simulink model "affine_single_integrator_ex"  (R2020b)
settings: Solver=ode4  StartTime=0.0  StopTime=50  FixedStep=0.01  RelTol=1e-3
InitFcn:
  | Initial_Parameters;
values from neighbouring files (symbols this model uses):
  cmd_sample = 0.1    [run_by_script.m]
  delay = 0.01    [Initial_Parameters.m]    (also in run_by_script.m)
  kalpha = 0.5    [Initial_Parameters.m]    (also in run_by_script.m)
  kbeta = 1.5    [Initial_Parameters.m]    (also in run_by_script.m = 0.5)
  kptheta = 100    [run_by_script.m]
  Kv = 0.987 / Tv    (= 6.16875)    [run_by_script.m]
  L = 10.5e-3    (= 0.0105)    [run_by_script.m]
  noise_p = normrnd(0.001, 0.03,[1 6])    [run_by_script.m]
  noise_pT = 3    [run_by_script.m]
  noise_v = normrnd(0.001, 0.03,[1 6])    [run_by_script.m]
  noise_vT = 0.1    [run_by_script.m]
  p = p(tout >= start_time, :)    [read_data.m]
  P0 = [2 0 ... (first row only)    [Initial_Parameters.m]    (also in run_by_script.m = [p(1,1:2:end)' p(2,2:2:end)'])
  R = 3.2e-3    (= 0.0032)    [run_by_script.m]
  seed_p = zeros(1,6)    [run_by_script.m]
  seed_v = zeros(1,6)    [run_by_script.m]
  stressMat = -fcn_StressMatrix(2,nodenum,m,P,neighborMat,fig_shape)    [Initial_Parameters.m]    (also in fcn_StressMatrix.m = -stressMat)
  tout = tout(tout >= start_time) - start_time    [read_data.m]    (also in run_by_script.m = out.tout)
  Tv = 0.16    [run_by_script.m]
  vl = 1    [run_by_script.m]
libraries: simulink x24
settings Model: Creator=Fitz  LastModifiedBy=xpp
settings OptimizationCC: BlockReduction=off  DefaultParameterBehavior=Inlined  BufferReuse=off
settings DebuggingCC: UnderSpecifiedDimensionMsg=warning

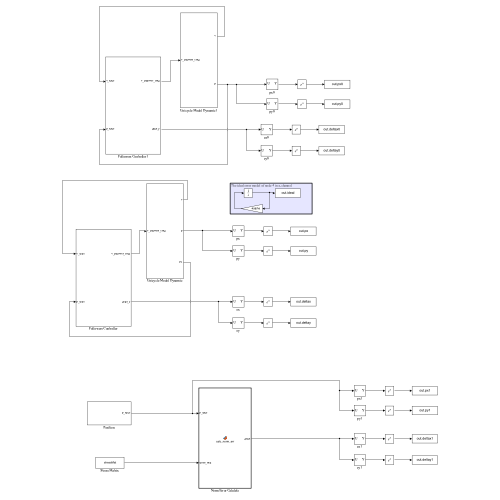
[thumbnail: Simulink's stored preview of the top-level diagram]
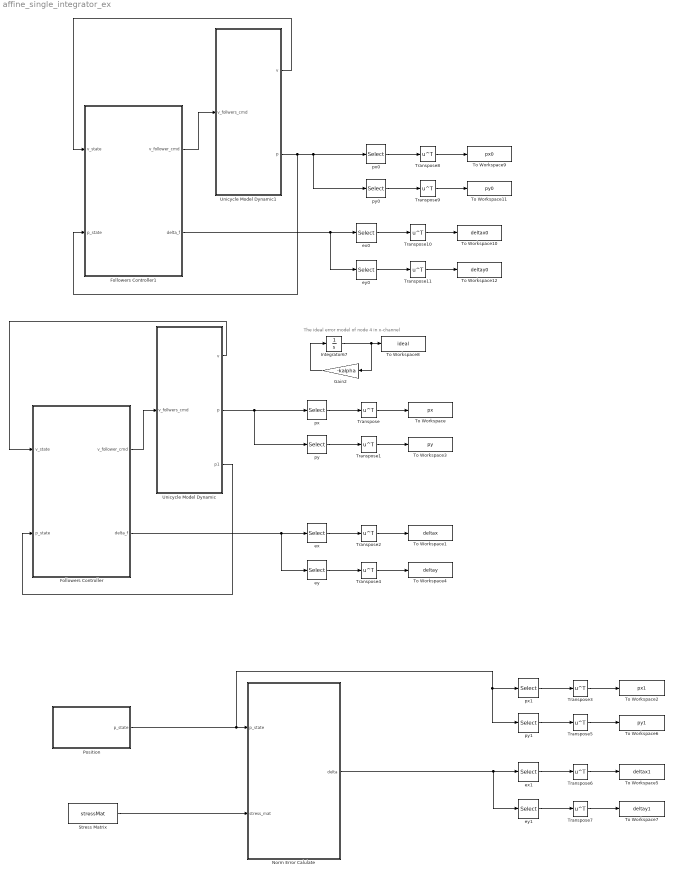
== system affine_single_integrator_ex ==
  note: The ideal error model of node 4 in x-channel
  Followers Controller : Subsystem
  Followers Controller1 : Subsystem
  Gain2 : Gain  Gain=-kalpha
  Integrator67 : Integrator  InitialCondition=P0(4,1)
  Norm Error Calulate : MATLAB Function  TreatAsAtomicUnit=on
  Position : Subsystem
  Stress Matrix : Constant  Value=stressMat
  To Workspace : ToWorkspace  VariableName=px  SampleTime=-1
      settings: Save2DSignal=2-D array (concatenate along first dimension)
  To Workspace1 : ToWorkspace  VariableName=deltax  SampleTime=-1
      settings: Save2DSignal=2-D array (concatenate along first dimension)
  To Workspace10 : ToWorkspace  VariableName=deltax0  SampleTime=-1
      settings: Save2DSignal=2-D array (concatenate along first dimension)
  To Workspace11 : ToWorkspace  VariableName=py0  SampleTime=-1
      settings: Save2DSignal=2-D array (concatenate along first dimension)
  To Workspace12 : ToWorkspace  VariableName=deltay0  SampleTime=-1
      settings: Save2DSignal=2-D array (concatenate along first dimension)
  To Workspace2 : ToWorkspace  VariableName=px1  SampleTime=-1
      settings: Save2DSignal=2-D array (concatenate along first dimension)
  To Workspace3 : ToWorkspace  VariableName=py  SampleTime=-1
      settings: Save2DSignal=2-D array (concatenate along first dimension)
  To Workspace4 : ToWorkspace  VariableName=deltay  SampleTime=-1
      settings: Save2DSignal=2-D array (concatenate along first dimension)
  To Workspace5 : ToWorkspace  VariableName=deltax1  SampleTime=-1
      settings: Save2DSignal=2-D array (concatenate along first dimension)
  To Workspace6 : ToWorkspace  VariableName=py1  SampleTime=-1
      settings: Save2DSignal=2-D array (concatenate along first dimension)
  To Workspace7 : ToWorkspace  VariableName=deltay1  SampleTime=-1
      settings: Save2DSignal=2-D array (concatenate along first dimension)
  To Workspace8 : ToWorkspace  VariableName=ideal  SampleTime=-1
      settings: Save2DSignal=2-D array (concatenate along first dimension)
  To Workspace9 : ToWorkspace  VariableName=px0  SampleTime=-1
      settings: Save2DSignal=2-D array (concatenate along first dimension)
  Transpose{,1..11} (12 alike) : Math  Operator=transpose  SaturateOnIntegerOverflow=on
  Unicycle Model Dynamic : Subsystem
  Unicycle Model Dynamic1 : Subsystem
  ex : Selector  NumberOfDimensions=2  InputPortWidth=3  IndexOptions=Select all,Index vector (dialog)  Indices=[1 3],1  OutputSizes=1,1
  ex0 : Selector  NumberOfDimensions=2  InputPortWidth=3  IndexOptions=Select all,Index vector (dialog)  Indices=[1 3],1  OutputSizes=1,1
  ex1 : Selector  NumberOfDimensions=2  InputPortWidth=3  IndexOptions=Select all,Index vector (dialog)  Indices=[1 3],1  OutputSizes=1,1
  ey : Selector  NumberOfDimensions=2  InputPortWidth=3  IndexOptions=Select all,Index vector (dialog)  Indices=[1 3],2  OutputSizes=1,1
  ey0 : Selector  NumberOfDimensions=2  InputPortWidth=3  IndexOptions=Select all,Index vector (dialog)  Indices=[1 3],2  OutputSizes=1,1
  ey1 : Selector  NumberOfDimensions=2  InputPortWidth=3  IndexOptions=Select all,Index vector (dialog)  Indices=[1 3],2  OutputSizes=1,1
  px : Selector  NumberOfDimensions=2  InputPortWidth=3  IndexOptions=Select all,Index vector (dialog)  Indices=[1 3],1  OutputSizes=1,1
  px0 : Selector  NumberOfDimensions=2  InputPortWidth=3  IndexOptions=Select all,Index vector (dialog)  Indices=[1 3],1  OutputSizes=1,1
  px1 : Selector  NumberOfDimensions=2  InputPortWidth=3  IndexOptions=Select all,Index vector (dialog)  Indices=[1 3],1  OutputSizes=1,1
  py : Selector  NumberOfDimensions=2  InputPortWidth=3  IndexOptions=Select all,Index vector (dialog)  Indices=[1 3],2  OutputSizes=1,1
  py0 : Selector  NumberOfDimensions=2  InputPortWidth=3  IndexOptions=Select all,Index vector (dialog)  Indices=[1 3],2  OutputSizes=1,1
  py1 : Selector  NumberOfDimensions=2  InputPortWidth=3  IndexOptions=Select all,Index vector (dialog)  Indices=[1 3],2  OutputSizes=1,1
  wires:
  Followers Controller/1(v_follower_cmd) -> Unicycle Model Dynamic/1(v_follwers_cmd)
  Unicycle Model Dynamic/2(p) -> px/1, py/1
  Followers Controller/2(delta_f) -> ex/1, ey/1
  ex/1 -> Transpose2/1
  py/1 -> Transpose1/1
  px/1 -> Transpose/1
  Transpose/1 -> To Workspace/1
  Transpose1/1 -> To Workspace3/1
  Transpose2/1 -> To Workspace1/1
  ey/1 -> Transpose4/1
  Transpose4/1 -> To Workspace4/1
  Gain2/1 -> Integrator67/1
  Integrator67/1 -> To Workspace8/1, Gain2/1
  Stress Matrix/1 -> Norm Error Calulate/2(stress_mat)
  py1/1 -> Transpose5/1
  Transpose6/1 -> To Workspace5/1
  px1/1 -> Transpose3/1
  Norm Error Calulate/1(delta) -> ex1/1, ey1/1
  Transpose3/1 -> To Workspace2/1
  Transpose7/1 -> To Workspace7/1
  Transpose5/1 -> To Workspace6/1
  ey1/1 -> Transpose7/1
  ex1/1 -> Transpose6/1
  Position/1(p_state) -> py1/1, px1/1, Norm Error Calulate/1(p_state)
  Followers Controller1/1(v_follower_cmd) -> Unicycle Model Dynamic1/1(v_follwers_cmd)
  Transpose9/1 -> To Workspace11/1
  ex0/1 -> Transpose10/1
  Followers Controller1/2(delta_f) -> ex0/1, ey0/1
  Transpose11/1 -> To Workspace12/1
  py0/1 -> Transpose9/1
  Transpose8/1 -> To Workspace9/1
  px0/1 -> Transpose8/1
  Transpose10/1 -> To Workspace10/1
  ey0/1 -> Transpose11/1
  Unicycle Model Dynamic/1(v) -> Followers Controller/1(v_state)
  Unicycle Model Dynamic/3(p1) -> Followers Controller/2(p_state)
  Unicycle Model Dynamic1/2(p) -> Followers Controller1/2(p_state), px0/1, py0/1
  Unicycle Model Dynamic1/1(v) -> Followers Controller1/1(v_state)

== system affine_single_integrator_ex/Followers Controller ==
  v_state : Inport
  p_state : Inport  Port=2
  Formation Controller : MATLAB Function  TreatAsAtomicUnit=on
  Kbeta : Constant  Value=kbeta
  Kp : Constant  Value=kalpha
  Stress Matrix : Constant  Value=stressMat
  Time Delay : VariableTransportDelay  MaximumDelay=10
  Zero-Order Hold : ZeroOrderHold  SampleTime=cmd_sample
  delay constant : Constant  Value=delay
  v_follower_cmd : Outport
  delta_f : Outport  Port=2
  wires:
  delay constant/1 -> Time Delay/2
  v_state/1 -> Time Delay/1
  p_state/1 -> Formation Controller/2(p_state)
  Stress Matrix/1 -> Formation Controller/3(stress_mat)
  Kbeta/1 -> Formation Controller/5(kbeta)
  Kp/1 -> Formation Controller/4(kalpha)
  Formation Controller/2(delta) -> delta_f/1
  Time Delay/1 -> Formation Controller/1(v_state)
  Formation Controller/1(v_cmd) -> Zero-Order Hold/1
  Zero-Order Hold/1 -> v_follower_cmd/1

== system affine_single_integrator_ex/Followers Controller1 ==
  v_state : Inport
  p_state : Inport  Port=2
  Formation Controller : MATLAB Function  TreatAsAtomicUnit=on
  Kbeta : Constant  Value=kbeta
  Kp : Constant  Value=kalpha
  Stress Matrix : Constant  Value=stressMat
  Time Delay : VariableTransportDelay  MaximumDelay=10
  Zero-Order Hold : ZeroOrderHold  SampleTime=cmd_sample
  delay constant : Constant  Value=delay
  v_follower_cmd : Outport
  delta_f : Outport  Port=2
  wires:
  delay constant/1 -> Time Delay/2
  v_state/1 -> Time Delay/1
  p_state/1 -> Formation Controller/2(p_state)
  Stress Matrix/1 -> Formation Controller/3(stress_mat)
  Kbeta/1 -> Formation Controller/5(kbeta)
  Kp/1 -> Formation Controller/4(kalpha)
  Formation Controller/2(delta) -> delta_f/1
  Time Delay/1 -> Formation Controller/1(v_state)
  Formation Controller/1(v_cmd) -> Zero-Order Hold/1
  Zero-Order Hold/1 -> v_follower_cmd/1

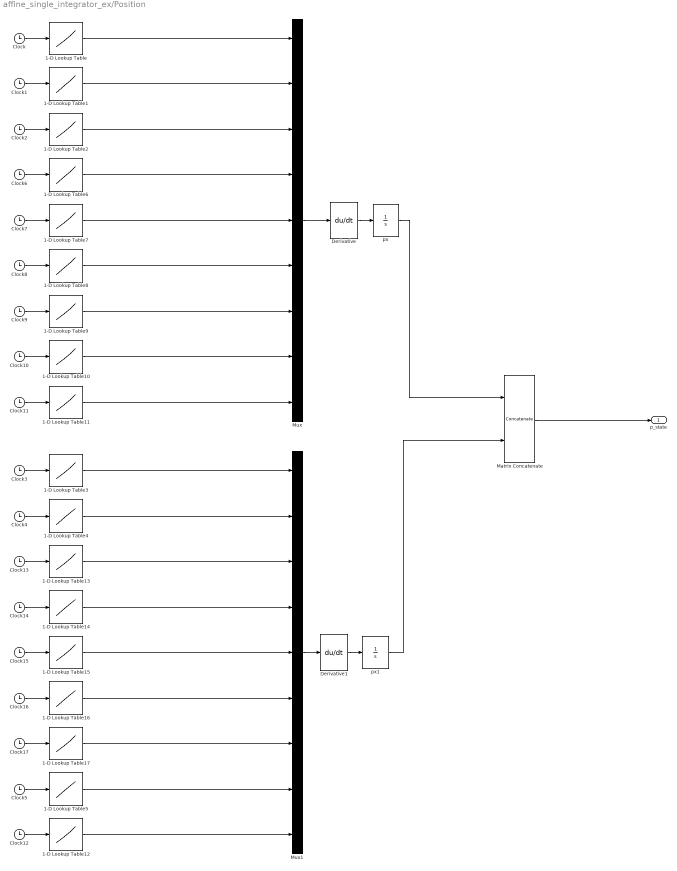
== system affine_single_integrator_ex/Position ==
  1-D Lookup Table : Lookup_n-D  NumberOfTableDimensions=1  BreakpointsForDimension1=tout  Table=p(:,1)  InternalRulePriority=Speed  RndMeth=Simplest  InputSameDT=on
  1-D Lookup Table1 : Lookup_n-D  NumberOfTableDimensions=1  BreakpointsForDimension1=tout  Table=p(:,3)  InternalRulePriority=Speed  RndMeth=Simplest  InputSameDT=on
  1-D Lookup Table10 : Lookup_n-D  NumberOfTableDimensions=1  BreakpointsForDimension1=tout  Table=p(:,15)  InternalRulePriority=Speed  RndMeth=Simplest  InputSameDT=on
  1-D Lookup Table11 : Lookup_n-D  NumberOfTableDimensions=1  BreakpointsForDimension1=tout  Table=p(:,17)  InternalRulePriority=Speed  RndMeth=Simplest  InputSameDT=on
  1-D Lookup Table12 : Lookup_n-D  NumberOfTableDimensions=1  BreakpointsForDimension1=tout  Table=p(:,18)  InternalRulePriority=Speed  RndMeth=Simplest  InputSameDT=on
  1-D Lookup Table13 : Lookup_n-D  NumberOfTableDimensions=1  BreakpointsForDimension1=tout  Table=p(:,6)  InternalRulePriority=Speed  RndMeth=Simplest  InputSameDT=on
  1-D Lookup Table14 : Lookup_n-D  NumberOfTableDimensions=1  BreakpointsForDimension1=tout  Table=p(:,8)  InternalRulePriority=Speed  RndMeth=Simplest  InputSameDT=on
  1-D Lookup Table15 : Lookup_n-D  NumberOfTableDimensions=1  BreakpointsForDimension1=tout  Table=p(:,10)  InternalRulePriority=Speed  RndMeth=Simplest  InputSameDT=on
  1-D Lookup Table16 : Lookup_n-D  NumberOfTableDimensions=1  BreakpointsForDimension1=tout  Table=p(:,12)  InternalRulePriority=Speed  RndMeth=Simplest  InputSameDT=on
  1-D Lookup Table17 : Lookup_n-D  NumberOfTableDimensions=1  BreakpointsForDimension1=tout  Table=p(:,14)  InternalRulePriority=Speed  RndMeth=Simplest  InputSameDT=on
  1-D Lookup Table2 : Lookup_n-D  NumberOfTableDimensions=1  BreakpointsForDimension1=tout  Table=p(:,5)  InternalRulePriority=Speed  RndMeth=Simplest  InputSameDT=on
  1-D Lookup Table3 : Lookup_n-D  NumberOfTableDimensions=1  BreakpointsForDimension1=tout  Table=p(:,2)  InternalRulePriority=Speed  RndMeth=Simplest  InputSameDT=on
  1-D Lookup Table4 : Lookup_n-D  NumberOfTableDimensions=1  BreakpointsForDimension1=tout  Table=p(:,4)  InternalRulePriority=Speed  RndMeth=Simplest  InputSameDT=on
  1-D Lookup Table5 : Lookup_n-D  NumberOfTableDimensions=1  BreakpointsForDimension1=tout  Table=p(:,16)  InternalRulePriority=Speed  RndMeth=Simplest  InputSameDT=on
  1-D Lookup Table6 : Lookup_n-D  NumberOfTableDimensions=1  BreakpointsForDimension1=tout  Table=p(:,7)  InternalRulePriority=Speed  RndMeth=Simplest  InputSameDT=on
  1-D Lookup Table7 : Lookup_n-D  NumberOfTableDimensions=1  BreakpointsForDimension1=tout  Table=p(:,9)  InternalRulePriority=Speed  RndMeth=Simplest  InputSameDT=on
  1-D Lookup Table8 : Lookup_n-D  NumberOfTableDimensions=1  BreakpointsForDimension1=tout  Table=p(:,11)  InternalRulePriority=Speed  RndMeth=Simplest  InputSameDT=on
  1-D Lookup Table9 : Lookup_n-D  NumberOfTableDimensions=1  BreakpointsForDimension1=tout  Table=p(:,13)  InternalRulePriority=Speed  RndMeth=Simplest  InputSameDT=on
  Clock{,1..17} (18 alike) : Clock
  Derivative : Derivative
  Derivative1 : Derivative
  Matrix Concatenate : Concatenate  Mode=Multidimensional array  ConcatenateDimension=2
  Mux : Mux  Inputs=9
  Mux1 : Mux  Inputs=9
  px : Integrator  InitialCondition=P0(:,1)
  px1 : Integrator  InitialCondition=P0(:,2)
  p_state : Outport
  wires:
  Clock/1 -> 1-D Lookup Table/1
  Clock1/1 -> 1-D Lookup Table1/1
  Clock2/1 -> 1-D Lookup Table2/1
  1-D Lookup Table1/1 -> Mux/2
  1-D Lookup Table/1 -> Mux/1
  1-D Lookup Table2/1 -> Mux/3
  Matrix Concatenate/1 -> p_state/1
  Mux/1 -> Derivative/1
  Clock8/1 -> 1-D Lookup Table8/1
  Clock7/1 -> 1-D Lookup Table7/1
  Clock6/1 -> 1-D Lookup Table6/1
  Clock11/1 -> 1-D Lookup Table11/1
  Clock10/1 -> 1-D Lookup Table10/1
  Clock9/1 -> 1-D Lookup Table9/1
  1-D Lookup Table11/1 -> Mux/9
  1-D Lookup Table10/1 -> Mux/8
  1-D Lookup Table9/1 -> Mux/7
  1-D Lookup Table8/1 -> Mux/6
  1-D Lookup Table7/1 -> Mux/5
  1-D Lookup Table6/1 -> Mux/4
  1-D Lookup Table16/1 -> Mux1/6
  1-D Lookup Table13/1 -> Mux1/3
  1-D Lookup Table17/1 -> Mux1/7
  1-D Lookup Table5/1 -> Mux1/8
  1-D Lookup Table15/1 -> Mux1/5
  Clock15/1 -> 1-D Lookup Table15/1
  1-D Lookup Table4/1 -> Mux1/2
  1-D Lookup Table14/1 -> Mux1/4
  1-D Lookup Table3/1 -> Mux1/1
  Clock14/1 -> 1-D Lookup Table14/1
  Clock12/1 -> 1-D Lookup Table12/1
  Clock13/1 -> 1-D Lookup Table13/1
  Clock17/1 -> 1-D Lookup Table17/1
  Clock4/1 -> 1-D Lookup Table4/1
  Clock3/1 -> 1-D Lookup Table3/1
  1-D Lookup Table12/1 -> Mux1/9
  Clock16/1 -> 1-D Lookup Table16/1
  Clock5/1 -> 1-D Lookup Table5/1
  Mux1/1 -> Derivative1/1
  Derivative/1 -> px/1
  px/1 -> Matrix Concatenate/1
  px1/1 -> Matrix Concatenate/2
  Derivative1/1 -> px1/1

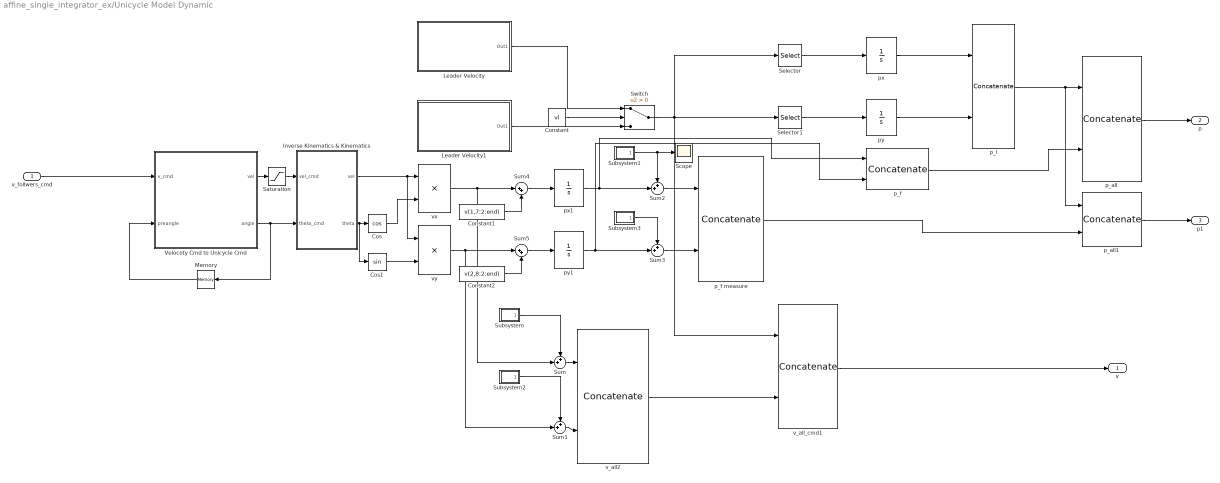
== system affine_single_integrator_ex/Unicycle Model Dynamic ==
  v_follwers_cmd : Inport
  Constant : Constant  Value=vl
  Constant1 : Constant  Value=v(1,7:2:end)
  Constant2 : Constant  Value=v(2,8:2:end)
  Cos : Trigonometry  Operator=cos
  Cos1 : Trigonometry
  Inverse Kinematics & Kinematics : Subsystem
  Leader Velocity : Subsystem
  Leader Velocity1 : Subsystem
  Memory : Memory
  Saturation : Saturate  UpperLimit=0.1  LowerLimit=0
  Scope : Scope
  Selector : Selector  NumberOfDimensions=2  InputPortWidth=3  IndexOptions=Select all,Index vector (dialog)  Indices=[1 3],1  OutputSizes=1,1
  Selector1 : Selector  NumberOfDimensions=2  InputPortWidth=3  IndexOptions=Select all,Index vector (dialog)  Indices=[1 3],2  OutputSizes=1,1
  Subsystem : Subsystem
  Subsystem1 : Subsystem
  Subsystem2 : Subsystem
  Subsystem3 : Subsystem
  Sum{,1..3} (4 alike) : Sum  Inputs=++|
  Sum4 : Sum  Inputs=|++
  Sum5 : Sum  Inputs=|++
  Switch : Switch  Criteria=u2 > Threshold
  Velocoty Cmd to Unicycle Cmd : MATLAB Function  TreatAsAtomicUnit=on
  p_all : Concatenate  Mode=Multidimensional array
  p_all1 : Concatenate  Mode=Multidimensional array
  p_f : Concatenate  Mode=Multidimensional array  ConcatenateDimension=2
  p_f measure : Concatenate  Mode=Multidimensional array  ConcatenateDimension=2
  p_l : Concatenate  Mode=Multidimensional array  ConcatenateDimension=2
  px : Integrator  InitialCondition=P0(1:3,1)
  px1 : Integrator  InitialCondition=P0(4:end,1)
  py : Integrator  InitialCondition=P0(1:3,2)
  py1 : Integrator  InitialCondition=P0(4:end,2)
  v_all2 : Concatenate  Mode=Multidimensional array  ConcatenateDimension=2
  v_all_cmd1 : Concatenate  Mode=Multidimensional array
  vx : Product
  vy : Product
  v : Outport
  p : Outport  Port=2
  p1 : Outport  Port=3
  wires:
  v_follwers_cmd/1 -> Velocoty Cmd to Unicycle Cmd/1(v_cmd)
  Memory/1 -> Velocoty Cmd to Unicycle Cmd/2(preangle)
  Cos/1 -> vx/2
  Cos1/1 -> vy/2
  Selector1/1 -> py/1
  Selector/1 -> px/1
  Switch/1 -> Selector/1, Selector1/1, v_all_cmd1/1
  Leader Velocity1/1(Out1) -> Switch/3
  Leader Velocity/1(Out1) -> Switch/1
  Constant/1 -> Switch/2
  vx/1 -> Sum4/1, Sum/2
  Velocoty Cmd to Unicycle Cmd/2(angle) -> Inverse Kinematics & Kinematics/2(theta_cmd), Memory/1
  vy/1 -> Sum5/1, Sum1/2
  Sum/1 -> v_all2/1
  Sum1/1 -> v_all2/2
  v_all2/1 -> v_all_cmd1/2
  v_all_cmd1/1 -> v/1
  Subsystem/1(Out1) -> Sum/1
  Subsystem2/1(Out1) -> Sum1/1
  px/1 -> p_l/1
  py/1 -> p_l/2
  px1/1 -> p_f/1, Sum2/2
  Subsystem1/1(Out1) -> Scope/1, Sum2/1
  py1/1 -> p_f/2, Sum3/2
  Subsystem3/1(Out1) -> Sum3/1
  Sum3/1 -> p_f measure/2
  Sum2/1 -> p_f measure/1
  p_l/1 -> p_all1/1, p_all/1
  p_f/1 -> p_all/2
  p_all/1 -> p/1
  p_f measure/1 -> p_all1/2
  p_all1/1 -> p1/1
  Constant1/1 -> Sum4/2
  Sum4/1 -> px1/1
  Constant2/1 -> Sum5/2
  Sum5/1 -> py1/1
  Velocoty Cmd to Unicycle Cmd/1(vel) -> Saturation/1
  Inverse Kinematics & Kinematics/1(vel) -> vy/1, vx/1
  Saturation/1 -> Inverse Kinematics & Kinematics/1(vel_cmd)
  Inverse Kinematics & Kinematics/2(theta) -> Cos1/1, Cos/1

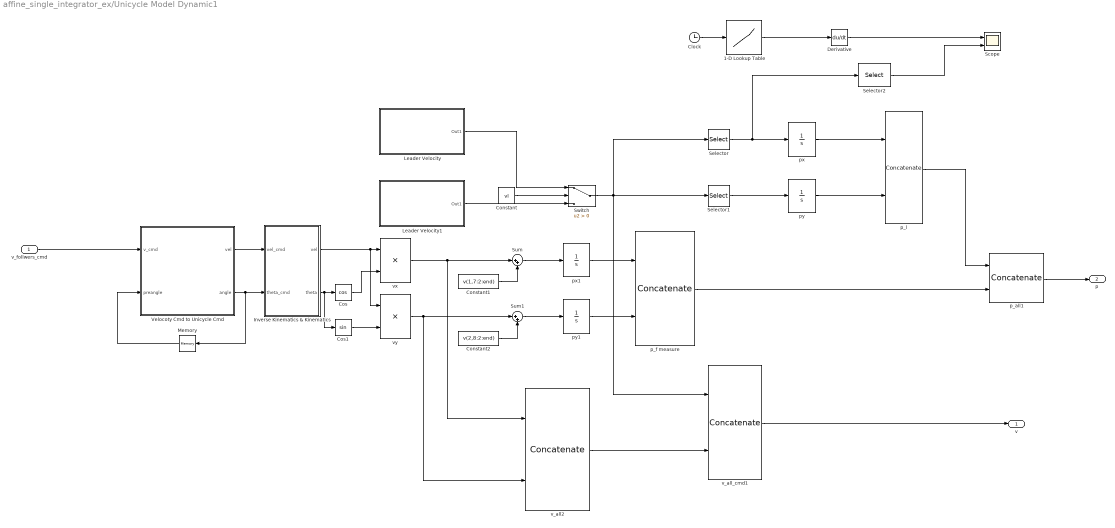
== system affine_single_integrator_ex/Unicycle Model Dynamic1 ==
  v_follwers_cmd : Inport
  1-D Lookup Table : Lookup_n-D  NumberOfTableDimensions=1  BreakpointsForDimension1=tout  Table=p(:,1)  InternalRulePriority=Speed  RndMeth=Simplest  InputSameDT=on
  Clock : Clock
  Constant : Constant  Value=vl
  Constant1 : Constant  Value=v(1,7:2:end)
  Constant2 : Constant  Value=v(2,8:2:end)
  Cos : Trigonometry  Operator=cos
  Cos1 : Trigonometry
  Derivative : Derivative
  Inverse Kinematics & Kinematics : Subsystem
  Leader Velocity : Subsystem
  Leader Velocity1 : Subsystem
  Memory : Memory
  Scope : Scope  NumInputPorts=2
  Selector : Selector  NumberOfDimensions=2  InputPortWidth=3  IndexOptions=Select all,Index vector (dialog)  Indices=[1 3],1  OutputSizes=1,1
  Selector1 : Selector  NumberOfDimensions=2  InputPortWidth=3  IndexOptions=Select all,Index vector (dialog)  Indices=[1 3],2  OutputSizes=1,1
  Selector2 : Selector  InputPortWidth=3  IndexOptions=Index vector (dialog)  Indices=1  OutputSizes=1
  Sum : Sum  Inputs=|++
  Sum1 : Sum  Inputs=|++
  Switch : Switch  Criteria=u2 > Threshold
  Velocoty Cmd to Unicycle Cmd : MATLAB Function  TreatAsAtomicUnit=on
  p_all1 : Concatenate  Mode=Multidimensional array
  p_f measure : Concatenate  Mode=Multidimensional array  ConcatenateDimension=2
  p_l : Concatenate  Mode=Multidimensional array  ConcatenateDimension=2
  px : Integrator  InitialCondition=P0(1:3,1)
  px1 : Integrator  InitialCondition=P0(4:end,1)
  py : Integrator  InitialCondition=P0(1:3,2)
  py1 : Integrator  InitialCondition=P0(4:end,2)
  v_all2 : Concatenate  Mode=Multidimensional array  ConcatenateDimension=2
  v_all_cmd1 : Concatenate  Mode=Multidimensional array
  vx : Product
  vy : Product
  v : Outport
  p : Outport  Port=2
  wires:
  v_follwers_cmd/1 -> Velocoty Cmd to Unicycle Cmd/1(v_cmd)
  Memory/1 -> Velocoty Cmd to Unicycle Cmd/2(preangle)
  Cos/1 -> vx/2
  Cos1/1 -> vy/2
  Selector1/1 -> py/1
  Selector/1 -> Selector2/1, px/1
  Switch/1 -> Selector/1, Selector1/1, v_all_cmd1/1
  Leader Velocity1/1(Out1) -> Switch/3
  Leader Velocity/1(Out1) -> Switch/1
  Constant/1 -> Switch/2
  Velocoty Cmd to Unicycle Cmd/2(angle) -> Inverse Kinematics & Kinematics/2(theta_cmd), Memory/1
  vx/1 -> Sum/1, v_all2/1
  v_all2/1 -> v_all_cmd1/2
  v_all_cmd1/1 -> v/1
  px/1 -> p_l/1
  py/1 -> p_l/2
  px1/1 -> p_f measure/1
  p_l/1 -> p_all1/1
  p_all1/1 -> p/1
  p_f measure/1 -> p_all1/2
  py1/1 -> p_f measure/2
  vy/1 -> Sum1/1, v_all2/2
  Clock/1 -> 1-D Lookup Table/1
  1-D Lookup Table/1 -> Derivative/1
  Selector2/1 -> Scope/2
  Derivative/1 -> Scope/1
  Sum/1 -> px1/1
  Constant1/1 -> Sum/2
  Constant2/1 -> Sum1/2
  Sum1/1 -> py1/1
  Inverse Kinematics & Kinematics/2(theta) -> Cos1/1, Cos/1
  Inverse Kinematics & Kinematics/1(vel) -> vy/1, vx/1
  Velocoty Cmd to Unicycle Cmd/1(vel) -> Inverse Kinematics & Kinematics/1(vel_cmd)

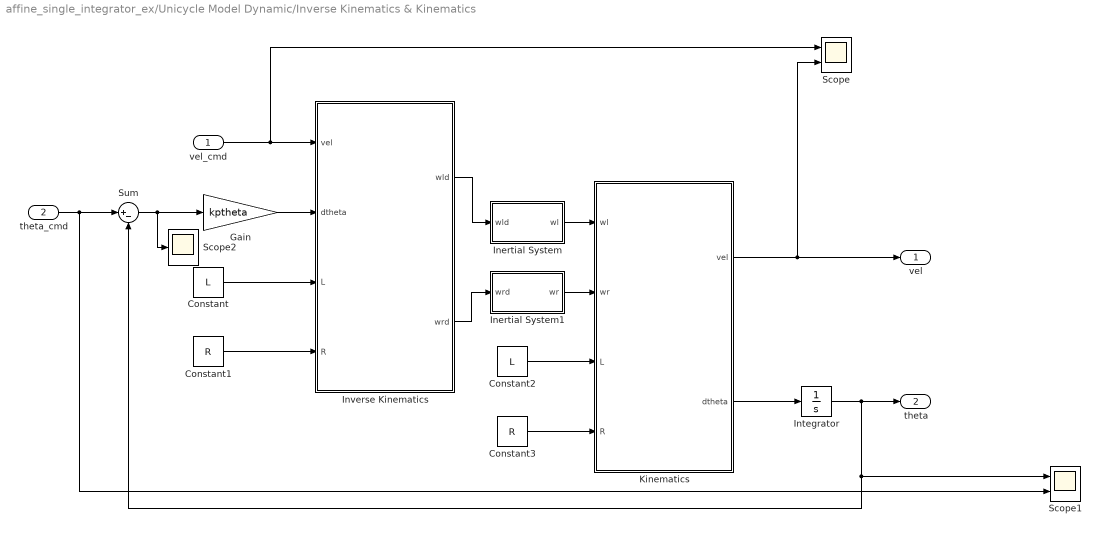
== system affine_single_integrator_ex/Unicycle Model Dynamic/Inverse Kinematics & Kinematics ==
  vel_cmd : Inport
  theta_cmd : Inport  Port=2
  Constant : Constant  Value=L
  Constant1 : Constant  Value=R
  Constant2 : Constant  Value=L
  Constant3 : Constant  Value=R
  Gain : Gain  Gain=kptheta
  Inertial System : Subsystem
  Inertial System1 : Subsystem
  Integrator : Integrator
  Inverse Kinematics : MATLAB Function  TreatAsAtomicUnit=on
  Kinematics : MATLAB Function  TreatAsAtomicUnit=on
  Scope : Scope  NumInputPorts=2
  Scope1 : Scope  NumInputPorts=2
  Scope2 : Scope
  Sum : Sum  Inputs=|+-
  vel : Outport
  theta : Outport  Port=2
  wires:
  vel_cmd/1 -> Scope/1, Inverse Kinematics/1(vel)
  Constant/1 -> Inverse Kinematics/3(L)
  Constant1/1 -> Inverse Kinematics/4(R)
  Constant3/1 -> Kinematics/4(R)
  Constant2/1 -> Kinematics/3(L)
  Integrator/1 -> Scope1/1, Sum/2, theta/1
  Kinematics/2(dtheta) -> Integrator/1
  Gain/1 -> Inverse Kinematics/2(dtheta)
  Sum/1 -> Scope2/1, Gain/1
  theta_cmd/1 -> Scope1/2, Sum/1
  Kinematics/1(vel) -> Scope/2, vel/1
  Inertial System1/1(wr) -> Kinematics/2(wr)
  Inertial System/1(wl) -> Kinematics/1(wl)
  Inverse Kinematics/1(wld) -> Inertial System/1(wld)
  Inverse Kinematics/2(wrd) -> Inertial System1/1(wrd)

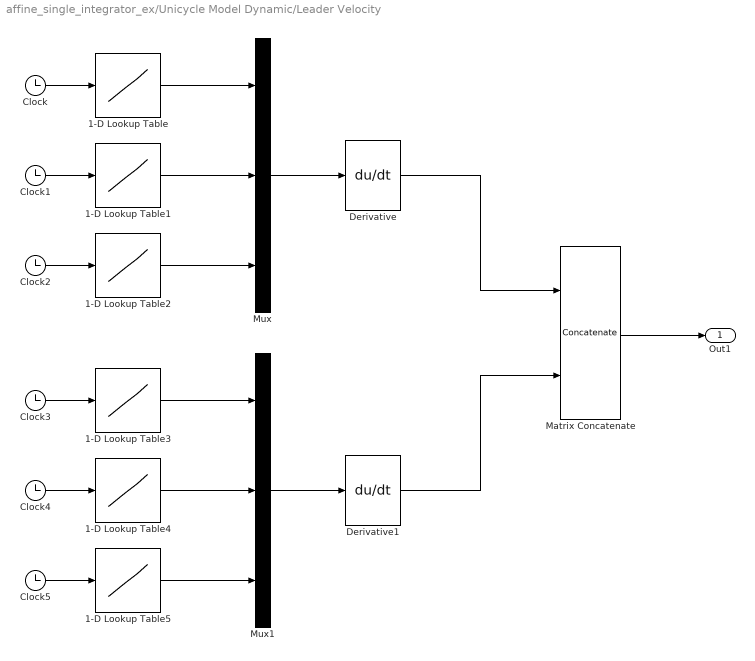
== system affine_single_integrator_ex/Unicycle Model Dynamic/Leader Velocity ==
  1-D Lookup Table : Lookup_n-D  NumberOfTableDimensions=1  BreakpointsForDimension1=tout  Table=p(:,1)  InternalRulePriority=Speed  RndMeth=Simplest  InputSameDT=on
  1-D Lookup Table1 : Lookup_n-D  NumberOfTableDimensions=1  BreakpointsForDimension1=tout  Table=p(:,3)  InternalRulePriority=Speed  RndMeth=Simplest  InputSameDT=on
  1-D Lookup Table2 : Lookup_n-D  NumberOfTableDimensions=1  BreakpointsForDimension1=tout  Table=p(:,5)  InternalRulePriority=Speed  RndMeth=Simplest  InputSameDT=on
  1-D Lookup Table3 : Lookup_n-D  NumberOfTableDimensions=1  BreakpointsForDimension1=tout  Table=p(:,2)  InternalRulePriority=Speed  RndMeth=Simplest  InputSameDT=on
  1-D Lookup Table4 : Lookup_n-D  NumberOfTableDimensions=1  BreakpointsForDimension1=tout  Table=p(:,4)  InternalRulePriority=Speed  RndMeth=Simplest  InputSameDT=on
  1-D Lookup Table5 : Lookup_n-D  NumberOfTableDimensions=1  BreakpointsForDimension1=tout  Table=p(:,6)  InternalRulePriority=Speed  RndMeth=Simplest  InputSameDT=on
  Clock{,1..5} (6 alike) : Clock
  Derivative : Derivative
  Derivative1 : Derivative
  Matrix Concatenate : Concatenate  Mode=Multidimensional array  ConcatenateDimension=2
  Mux : Mux  Inputs=3
  Mux1 : Mux  Inputs=3
  Out1 : Outport
  wires:
  Clock/1 -> 1-D Lookup Table/1
  Clock1/1 -> 1-D Lookup Table1/1
  Clock2/1 -> 1-D Lookup Table2/1
  Clock3/1 -> 1-D Lookup Table3/1
  Clock4/1 -> 1-D Lookup Table4/1
  Clock5/1 -> 1-D Lookup Table5/1
  1-D Lookup Table1/1 -> Mux/2
  1-D Lookup Table/1 -> Mux/1
  1-D Lookup Table2/1 -> Mux/3
  Mux/1 -> Derivative/1
  Mux1/1 -> Derivative1/1
  1-D Lookup Table4/1 -> Mux1/2
  1-D Lookup Table5/1 -> Mux1/3
  1-D Lookup Table3/1 -> Mux1/1
  Matrix Concatenate/1 -> Out1/1
  Derivative/1 -> Matrix Concatenate/1
  Derivative1/1 -> Matrix Concatenate/2

== system affine_single_integrator_ex/Unicycle Model Dynamic/Leader Velocity1 ==
  Constant{,1..5} (6 alike) : Constant  Value=0
  Matrix Concatenate : Concatenate  Mode=Multidimensional array  ConcatenateDimension=2
  Mux : Mux  Inputs=3
  Mux1 : Mux  Inputs=3
  Out1 : Outport
  wires:
  Constant1/1 -> Mux/2
  Constant/1 -> Mux/1
  Constant2/1 -> Mux/3
  Constant4/1 -> Mux1/2
  Constant5/1 -> Mux1/3
  Constant3/1 -> Mux1/1
  Matrix Concatenate/1 -> Out1/1
  Mux/1 -> Matrix Concatenate/1
  Mux1/1 -> Matrix Concatenate/2

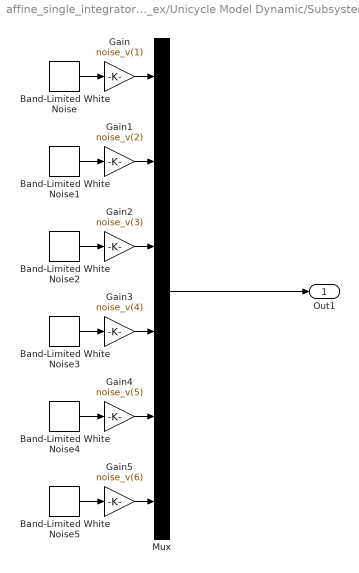
== system affine_single_integrator_ex/Unicycle Model Dynamic/Subsystem ==
  Band-Limited White Noise : simulink/Sources/Band-Limited White Noise  Cov=[0.01]  Ts=noise_vT  seed=seed_v(1)
  Band-Limited White Noise1 : simulink/Sources/Band-Limited White Noise  Cov=[0.01]  Ts=noise_vT  seed=seed_v(2)
  Band-Limited White Noise2 : simulink/Sources/Band-Limited White Noise  Cov=[0.01]  Ts=noise_vT  seed=seed_v(3)
  Band-Limited White Noise3 : simulink/Sources/Band-Limited White Noise  Cov=[0.01]  Ts=noise_vT  seed=seed_v(4)
  Band-Limited White Noise4 : simulink/Sources/Band-Limited White Noise  Cov=[0.01]  Ts=noise_vT  seed=seed_v(5)
  Band-Limited White Noise5 : simulink/Sources/Band-Limited White Noise  Cov=[0.01]  Ts=noise_vT  seed=seed_v(6)
  Gain : Gain  Gain=noise_v(1)
  Gain1 : Gain  Gain=noise_v(2)
  Gain2 : Gain  Gain=noise_v(3)
  Gain3 : Gain  Gain=noise_v(4)
  Gain4 : Gain  Gain=noise_v(5)
  Gain5 : Gain  Gain=noise_v(6)
  Mux : Mux  Inputs=6
  Out1 : Outport
  wires:
  Band-Limited White Noise5/1 -> Gain5/1
  Band-Limited White Noise4/1 -> Gain4/1
  Band-Limited White Noise3/1 -> Gain3/1
  Band-Limited White Noise2/1 -> Gain2/1
  Band-Limited White Noise1/1 -> Gain1/1
  Band-Limited White Noise/1 -> Gain/1
  Mux/1 -> Out1/1
  Gain/1 -> Mux/1
  Gain1/1 -> Mux/2
  Gain2/1 -> Mux/3
  Gain3/1 -> Mux/4
  Gain4/1 -> Mux/5
  Gain5/1 -> Mux/6

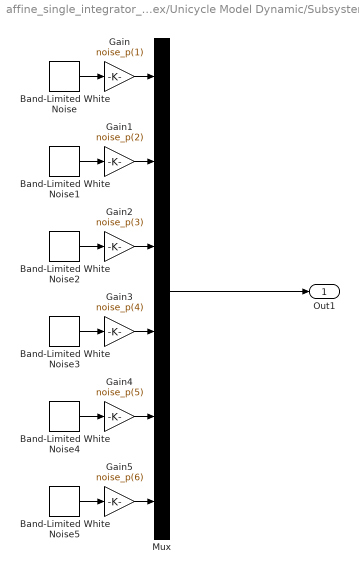
== system affine_single_integrator_ex/Unicycle Model Dynamic/Subsystem1 ==
  Band-Limited White Noise : simulink/Sources/Band-Limited White Noise  Cov=[0.01]  Ts=noise_pT  seed=seed_p(1)
  Band-Limited White Noise1 : simulink/Sources/Band-Limited White Noise  Cov=[0.01]  Ts=noise_pT  seed=seed_p(2)
  Band-Limited White Noise2 : simulink/Sources/Band-Limited White Noise  Cov=[0.01]  Ts=noise_pT  seed=seed_p(3)
  Band-Limited White Noise3 : simulink/Sources/Band-Limited White Noise  Cov=[0.01]  Ts=noise_pT  seed=seed_p(4)
  Band-Limited White Noise4 : simulink/Sources/Band-Limited White Noise  Cov=[0.01]  Ts=noise_pT  seed=seed_p(5)
  Band-Limited White Noise5 : simulink/Sources/Band-Limited White Noise  Cov=[0.01]  Ts=noise_pT  seed=seed_p(6)
  Gain : Gain  Gain=noise_p(1)
  Gain1 : Gain  Gain=noise_p(2)
  Gain2 : Gain  Gain=noise_p(3)
  Gain3 : Gain  Gain=noise_p(4)
  Gain4 : Gain  Gain=noise_p(5)
  Gain5 : Gain  Gain=noise_p(6)
  Mux : Mux  Inputs=6
  Out1 : Outport
  wires:
  Band-Limited White Noise5/1 -> Gain5/1
  Band-Limited White Noise4/1 -> Gain4/1
  Band-Limited White Noise3/1 -> Gain3/1
  Band-Limited White Noise2/1 -> Gain2/1
  Band-Limited White Noise1/1 -> Gain1/1
  Band-Limited White Noise/1 -> Gain/1
  Mux/1 -> Out1/1
  Gain/1 -> Mux/1
  Gain1/1 -> Mux/2
  Gain2/1 -> Mux/3
  Gain3/1 -> Mux/4
  Gain4/1 -> Mux/5
  Gain5/1 -> Mux/6

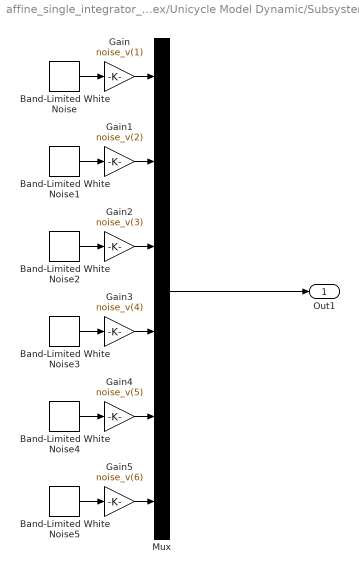
== system affine_single_integrator_ex/Unicycle Model Dynamic/Subsystem2 ==
  Band-Limited White Noise : simulink/Sources/Band-Limited White Noise  Cov=[0.01]  Ts=noise_vT  seed=seed_v(1)
  Band-Limited White Noise1 : simulink/Sources/Band-Limited White Noise  Cov=[0.01]  Ts=noise_vT  seed=seed_v(2)
  Band-Limited White Noise2 : simulink/Sources/Band-Limited White Noise  Cov=[0.01]  Ts=noise_vT  seed=seed_v(3)
  Band-Limited White Noise3 : simulink/Sources/Band-Limited White Noise  Cov=[0.01]  Ts=noise_vT  seed=seed_v(4)
  Band-Limited White Noise4 : simulink/Sources/Band-Limited White Noise  Cov=[0.01]  Ts=noise_vT  seed=seed_v(5)
  Band-Limited White Noise5 : simulink/Sources/Band-Limited White Noise  Cov=[0.01]  Ts=noise_vT  seed=seed_v(6)
  Gain : Gain  Gain=noise_v(1)
  Gain1 : Gain  Gain=noise_v(2)
  Gain2 : Gain  Gain=noise_v(3)
  Gain3 : Gain  Gain=noise_v(4)
  Gain4 : Gain  Gain=noise_v(5)
  Gain5 : Gain  Gain=noise_v(6)
  Mux : Mux  Inputs=6
  Out1 : Outport
  wires:
  Band-Limited White Noise5/1 -> Gain5/1
  Band-Limited White Noise4/1 -> Gain4/1
  Band-Limited White Noise3/1 -> Gain3/1
  Band-Limited White Noise2/1 -> Gain2/1
  Band-Limited White Noise1/1 -> Gain1/1
  Band-Limited White Noise/1 -> Gain/1
  Mux/1 -> Out1/1
  Gain/1 -> Mux/1
  Gain1/1 -> Mux/2
  Gain2/1 -> Mux/3
  Gain3/1 -> Mux/4
  Gain4/1 -> Mux/5
  Gain5/1 -> Mux/6

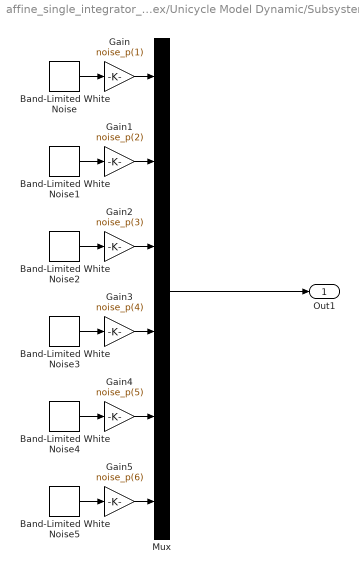
== system affine_single_integrator_ex/Unicycle Model Dynamic/Subsystem3 ==
  Band-Limited White Noise : simulink/Sources/Band-Limited White Noise  Cov=[0.01]  Ts=noise_pT  seed=seed_p(1)
  Band-Limited White Noise1 : simulink/Sources/Band-Limited White Noise  Cov=[0.01]  Ts=noise_pT  seed=seed_p(2)
  Band-Limited White Noise2 : simulink/Sources/Band-Limited White Noise  Cov=[0.01]  Ts=noise_pT  seed=seed_p(3)
  Band-Limited White Noise3 : simulink/Sources/Band-Limited White Noise  Cov=[0.01]  Ts=noise_pT  seed=seed_p(4)
  Band-Limited White Noise4 : simulink/Sources/Band-Limited White Noise  Cov=[0.01]  Ts=noise_pT  seed=seed_p(5)
  Band-Limited White Noise5 : simulink/Sources/Band-Limited White Noise  Cov=[0.01]  Ts=noise_pT  seed=seed_p(6)
  Gain : Gain  Gain=noise_p(1)
  Gain1 : Gain  Gain=noise_p(2)
  Gain2 : Gain  Gain=noise_p(3)
  Gain3 : Gain  Gain=noise_p(4)
  Gain4 : Gain  Gain=noise_p(5)
  Gain5 : Gain  Gain=noise_p(6)
  Mux : Mux  Inputs=6
  Out1 : Outport
  wires:
  Band-Limited White Noise5/1 -> Gain5/1
  Band-Limited White Noise4/1 -> Gain4/1
  Band-Limited White Noise3/1 -> Gain3/1
  Band-Limited White Noise2/1 -> Gain2/1
  Band-Limited White Noise1/1 -> Gain1/1
  Band-Limited White Noise/1 -> Gain/1
  Mux/1 -> Out1/1
  Gain/1 -> Mux/1
  Gain1/1 -> Mux/2
  Gain2/1 -> Mux/3
  Gain3/1 -> Mux/4
  Gain4/1 -> Mux/5
  Gain5/1 -> Mux/6

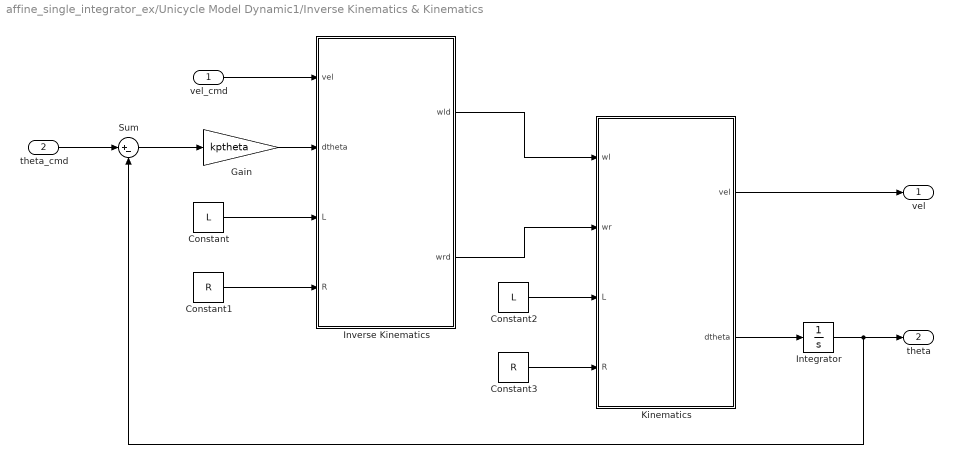
== system affine_single_integrator_ex/Unicycle Model Dynamic1/Inverse Kinematics & Kinematics ==
  vel_cmd : Inport
  theta_cmd : Inport  Port=2
  Constant : Constant  Value=L
  Constant1 : Constant  Value=R
  Constant2 : Constant  Value=L
  Constant3 : Constant  Value=R
  Gain : Gain  Gain=kptheta
  Integrator : Integrator
  Inverse Kinematics : MATLAB Function  TreatAsAtomicUnit=on
  Kinematics : MATLAB Function  TreatAsAtomicUnit=on
  Sum : Sum  Inputs=|+-
  vel : Outport
  theta : Outport  Port=2
  wires:
  vel_cmd/1 -> Inverse Kinematics/1(vel)
  Constant/1 -> Inverse Kinematics/3(L)
  Constant1/1 -> Inverse Kinematics/4(R)
  Inverse Kinematics/1(wld) -> Kinematics/1(wl)
  Inverse Kinematics/2(wrd) -> Kinematics/2(wr)
  Constant3/1 -> Kinematics/4(R)
  Constant2/1 -> Kinematics/3(L)
  Integrator/1 -> Sum/2, theta/1
  Kinematics/2(dtheta) -> Integrator/1
  Gain/1 -> Inverse Kinematics/2(dtheta)
  Sum/1 -> Gain/1
  theta_cmd/1 -> Sum/1
  Kinematics/1(vel) -> vel/1

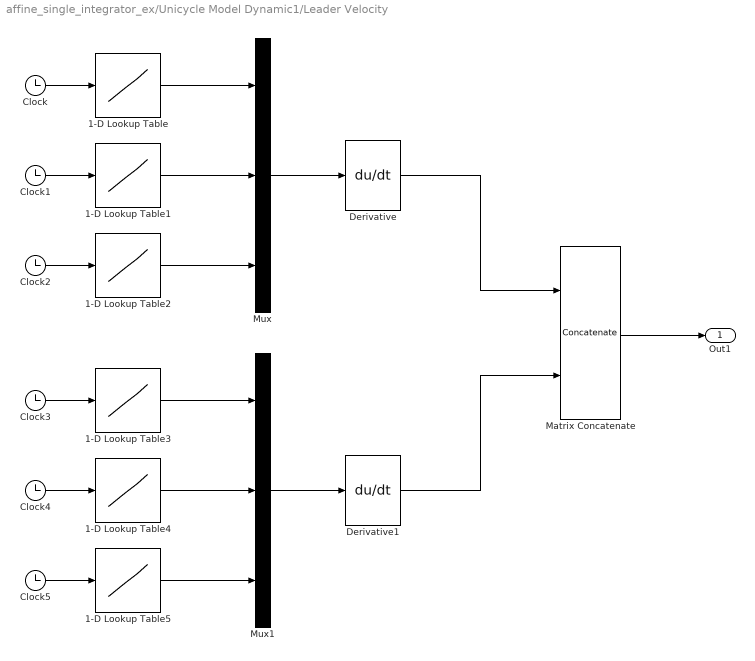
== system affine_single_integrator_ex/Unicycle Model Dynamic1/Leader Velocity ==
  1-D Lookup Table : Lookup_n-D  NumberOfTableDimensions=1  BreakpointsForDimension1=tout  Table=p(:,1)  InternalRulePriority=Speed  RndMeth=Simplest  InputSameDT=on
  1-D Lookup Table1 : Lookup_n-D  NumberOfTableDimensions=1  BreakpointsForDimension1=tout  Table=p(:,3)  InternalRulePriority=Speed  RndMeth=Simplest  InputSameDT=on
  1-D Lookup Table2 : Lookup_n-D  NumberOfTableDimensions=1  BreakpointsForDimension1=tout  Table=p(:,5)  InternalRulePriority=Speed  RndMeth=Simplest  InputSameDT=on
  1-D Lookup Table3 : Lookup_n-D  NumberOfTableDimensions=1  BreakpointsForDimension1=tout  Table=p(:,2)  InternalRulePriority=Speed  RndMeth=Simplest  InputSameDT=on
  1-D Lookup Table4 : Lookup_n-D  NumberOfTableDimensions=1  BreakpointsForDimension1=tout  Table=p(:,4)  InternalRulePriority=Speed  RndMeth=Simplest  InputSameDT=on
  1-D Lookup Table5 : Lookup_n-D  NumberOfTableDimensions=1  BreakpointsForDimension1=tout  Table=p(:,6)  InternalRulePriority=Speed  RndMeth=Simplest  InputSameDT=on
  Clock{,1..5} (6 alike) : Clock
  Derivative : Derivative
  Derivative1 : Derivative
  Matrix Concatenate : Concatenate  Mode=Multidimensional array  ConcatenateDimension=2
  Mux : Mux  Inputs=3
  Mux1 : Mux  Inputs=3
  Out1 : Outport
  wires:
  Clock/1 -> 1-D Lookup Table/1
  Clock1/1 -> 1-D Lookup Table1/1
  Clock2/1 -> 1-D Lookup Table2/1
  Clock3/1 -> 1-D Lookup Table3/1
  Clock4/1 -> 1-D Lookup Table4/1
  Clock5/1 -> 1-D Lookup Table5/1
  1-D Lookup Table1/1 -> Mux/2
  1-D Lookup Table/1 -> Mux/1
  1-D Lookup Table2/1 -> Mux/3
  Mux/1 -> Derivative/1
  Mux1/1 -> Derivative1/1
  1-D Lookup Table4/1 -> Mux1/2
  1-D Lookup Table5/1 -> Mux1/3
  1-D Lookup Table3/1 -> Mux1/1
  Matrix Concatenate/1 -> Out1/1
  Derivative/1 -> Matrix Concatenate/1
  Derivative1/1 -> Matrix Concatenate/2

== system affine_single_integrator_ex/Unicycle Model Dynamic1/Leader Velocity1 ==
  Constant{,1..5} (6 alike) : Constant  Value=0
  Matrix Concatenate : Concatenate  Mode=Multidimensional array  ConcatenateDimension=2
  Mux : Mux  Inputs=3
  Mux1 : Mux  Inputs=3
  Out1 : Outport
  wires:
  Constant1/1 -> Mux/2
  Constant/1 -> Mux/1
  Constant2/1 -> Mux/3
  Constant4/1 -> Mux1/2
  Constant5/1 -> Mux1/3
  Constant3/1 -> Mux1/1
  Matrix Concatenate/1 -> Out1/1
  Mux/1 -> Matrix Concatenate/1
  Mux1/1 -> Matrix Concatenate/2

== system affine_single_integrator_ex/Unicycle Model Dynamic/Inverse Kinematics & Kinematics/Inertial System ==
  wld : Inport
  Gain : Gain  Gain=Kv
  Gain1 : Gain  Gain=1/Tv
  Integrator : Integrator
  Sum : Sum  Inputs=|+-
  wl : Outport
  wires:
  wld/1 -> Gain/1
  Integrator/1 -> Gain1/1, wl/1
  Gain/1 -> Sum/1
  Sum/1 -> Integrator/1
  Gain1/1 -> Sum/2

== system affine_single_integrator_ex/Unicycle Model Dynamic/Inverse Kinematics & Kinematics/Inertial System1 ==
  wrd : Inport
  Gain : Gain  Gain=Kv
  Gain1 : Gain  Gain=1/Tv
  Integrator : Integrator
  Sum : Sum  Inputs=|+-
  wr : Outport
  wires:
  wrd/1 -> Gain/1
  Integrator/1 -> Gain1/1, wr/1
  Gain/1 -> Sum/1
  Sum/1 -> Integrator/1
  Gain1/1 -> Sum/2

== matlab function affine_single_integrator_ex/Unicycle Model Dynamic/Inverse Kinematics & Kinematics/Kinematics ==
  data: wl input; vel output; wr input; L input; R input; dtheta output
function [vel, dtheta] = Kinematics(wl, wr, L, R)
vel = R/2*(wl + wr);
dtheta = R*(wr - wl)/L;
end

== matlab function affine_single_integrator_ex/Norm Error Calulate ==
  data: p_state input; stress_mat input; delta output
function delta = calc_norm_err(p_state, stress_mat)
leaders_num = 3;
stressmat_ff = stress_mat(leaders_num+1:end,leaders_num+1:end);
stressmat_fl = stress_mat(leaders_num+1:end,1:leaders_num);
inv_stressmat_ff = inv(stressmat_ff);

delta = p_state(leaders_num+1:end,:) + inv_stressmat_ff * stressmat_fl * p_state(1:leaders_num,:);

== matlab function affine_single_integrator_ex/Unicycle Model Dynamic/Velocoty Cmd to Unicycle Cmd ==
  data: v_cmd input; vel output size=[followerNum, 1]; angle output size=[followerNum, 1]; preangle input
function [vel, angle] = fcn(v_cmd, preangle)
vel = 0.05 + zeros(size(v_cmd,1), 1);
angle = zeros(size(v_cmd,1), 1);

for i = 1:length(vel)
    Vx = v_cmd(i,1);
    Vy = v_cmd(i,2);
    vel(i) = sqrt(Vx^2+Vy^2);


    if Vx > 0 && Vy > 0
        angle(i) = atan(Vy/Vx);
    elseif Vx < 0 && Vy > 0
        angle(i) = pi+atan(Vy/Vx);
    elseif Vx < 0 && Vy < 0
        angle(i) = pi+atan(Vy/Vx);
    else
        angle(i) = 2*pi+atan(Vy/Vx);
    end

    if Vx == 0 && Vy > 0
        angle(i) = pi/2;
    end
    if Vx == 0 && Vy < 0
        angle(i) = -pi/2;
    end
    if Vx == 0 && Vy == 0
        angle(i) = preangle(i);
    end
    if Vy == 0 && Vx > 0
        angle(i) = 0;
    end
    if Vy == 0 && Vx < 0
        angle(i) = -pi;
    end

end

== matlab function affine_single_integrator_ex/Followers Controller1/Formation Controller ==
  data: v_state input; p_state input; stress_mat input; kalpha input; v_cmd output size=[followerNum, dim]; kbeta input; delta output
function [v_cmd, delta] = formation_controller(v_state, p_state, stress_mat, kalpha, kbeta)
leaders_num = 3;
stressmat_ff = stress_mat(leaders_num+1:end,leaders_num+1:end);
stressmat_fl = stress_mat(leaders_num+1:end,1:leaders_num);
inv_stressmat_ff = inv(stressmat_ff);

delta = p_state(leaders_num+1:end,:) + inv_stressmat_ff * stressmat_fl * p_state(1:leaders_num,:);
E = stressmat_fl * p_state(1:leaders_num,:) + stressmat_ff * p_state(leaders_num+1:end,:);
dE = stressmat_fl * v_state(1:leaders_num,:) + stressmat_ff * v_state(leaders_num+1:end,:);

v_cmd = v_state(leaders_num+1:end,:) - kbeta * (kalpha*E + dE);

== matlab function affine_single_integrator_ex/Followers Controller/Formation Controller ==
  data: v_state input; p_state input; stress_mat input; kalpha input; v_cmd output size=[followerNum, dim]; kbeta input; delta output
function [v_cmd, delta] = formation_controller(v_state, p_state, stress_mat, kalpha, kbeta)
leaders_num = 3;
stressmat_ff = stress_mat(leaders_num+1:end,leaders_num+1:end);
stressmat_fl = stress_mat(leaders_num+1:end,1:leaders_num);
inv_stressmat_ff = inv(stressmat_ff);

delta = p_state(leaders_num+1:end,:) + inv_stressmat_ff * stressmat_fl * p_state(1:leaders_num,:);
E = stressmat_fl * p_state(1:leaders_num,:) + stressmat_ff * p_state(leaders_num+1:end,:);
dE = stressmat_fl * v_state(1:leaders_num,:) + stressmat_ff * v_state(leaders_num+1:end,:);

v_cmd = v_state(leaders_num+1:end,:) - kbeta * (kalpha*E + dE);

== matlab function affine_single_integrator_ex/Unicycle Model Dynamic1/Velocoty Cmd to Unicycle Cmd ==
  data: v_cmd input; vel output size=[followerNum, 1]; angle output size=[followerNum, 1]; preangle input
function [vel, angle] = fcn(v_cmd, preangle)
vel = zeros(size(v_cmd,1), 1);
angle = zeros(size(v_cmd,1), 1);

for i = 1:length(vel)
    Vx = v_cmd(i,1);
    Vy = v_cmd(i,2);
    vel(i) = sqrt(Vx^2+Vy^2);


    if Vx > 0 && Vy > 0
        angle(i) = atan(Vy/Vx);
    elseif Vx < 0 && Vy > 0
        angle(i) = pi+atan(Vy/Vx);
    elseif Vx < 0 && Vy < 0
        angle(i) = pi+atan(Vy/Vx);
    else
        angle(i) = 2*pi+atan(Vy/Vx);
    end

    if Vx == 0 && Vy > 0
        angle(i) = pi/2;
    end
    if Vx == 0 && Vy < 0
        angle(i) = -pi/2;
    end
    if Vx == 0 && Vy == 0
        angle(i) = preangle(i);
    end
    if Vy == 0 && Vx > 0
        angle(i) = 0;
    end
    if Vy == 0 && Vx < 0
        angle(i) = -pi;
    end

    dangle = angle(i) - preangle(i);
    if dangle > pi
        angle(i) = angle(i) - 2*pi;
    end
    if dangle < -pi
        angle(i) = angle(i) + 2*pi;
    end
end

== matlab function affine_single_integrator_ex/Unicycle Model Dynamic1/Inverse Kinematics & Kinematics/Inverse Kinematics ==
  data: vel input; wld output; dtheta input; L input; R input; wrd output
function [wld, wrd] = InverseKinematics(vel, dtheta, L, R)
wrd = vel/R + L*dtheta/2/R;
wld = vel/R - L*dtheta/2/R;
end

== matlab function affine_single_integrator_ex/Unicycle Model Dynamic1/Inverse Kinematics & Kinematics/Kinematics ==
  data: wl input; vel output; wr input; L input; R input; dtheta output
function [vel, dtheta] = Kinematics(wl, wr, L, R)
vel = R/2*(wl + wr);
dtheta = R*(wr - wl)/L;
end

== matlab function affine_single_integrator_ex/Unicycle Model Dynamic/Inverse Kinematics & Kinematics/Inverse Kinematics ==
  data: vel input; wld output; dtheta input; L input; R input; wrd output
function [wld, wrd] = InverseKinematics(vel, dtheta, L, R)
wrd = vel/R + L*dtheta/2/R;
wld = vel/R - L*dtheta/2/R;
end
